simulink model "closedLoop"  (R2014b)
settings: Solver=ode45  StartTime=0.0  StopTime=inf  RelTol=1e-3
libraries: simulink x3, aerolibanimutils x1
settings Model: Creator=Owen  LastModifiedBy=Owen
settings SFSimCC: SimUserSources=TORCSLink.c
settings RTWCC: RTWUseSimCustomCode=on  CustomSource=TORCSLink.c

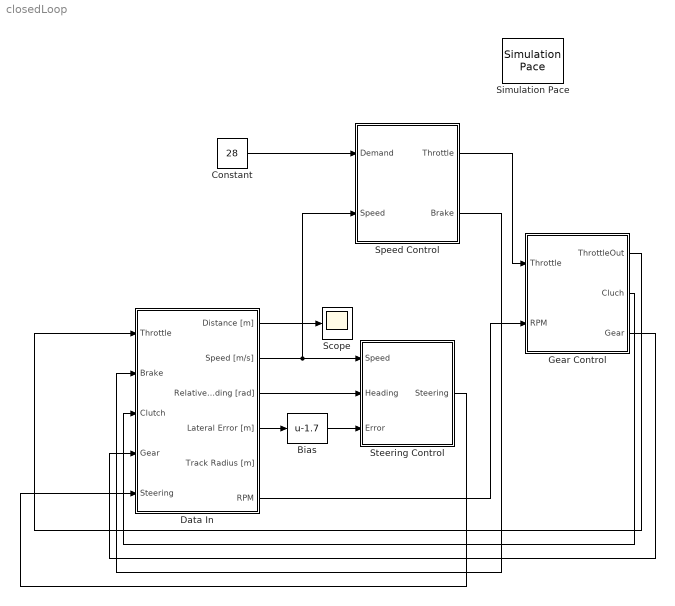
== system closedLoop ==
  Bias : Bias  Bias=-1.7
  Constant : Constant  Value=28  LockScale=on
  Data In : Subsystem
  Gear Control : Subsystem
  Scope : Scope
      settings: YMin=20250  YMax=20500  SaveName=ScopeData3
  Simulation Pace : aerolibanimutils/Simulation Pace  SimulationPace=1  SleepMode=MATLAB Thread  OutputPaceError=off  SampleTime=1/100
      settings: AttributesFormatString=%<SimulationPace> sec/sec
  Speed Control : Subsystem
  Steering Control : Subsystem
  wires:
  Data In/2(Speed [m/s]) -> Speed Control/2(Speed), Steering Control/1(Speed)
  Data In/3(Relative Heading [rad]) -> Steering Control/2(Heading)
  Data In/4(Lateral Error [m]) -> Bias/1
  Constant/1 -> Speed Control/1(Demand)
  Speed Control/1(Throttle) -> Gear Control/1(Throttle)
  Speed Control/2(Brake) -> Data In/2(Brake)
  Steering Control/1(Steering) -> Data In/5(Steering)
  Gear Control/1(ThrottleOut) -> Data In/1(Throttle)
  Gear Control/2(Cluch) -> Data In/3(Clutch)
  Gear Control/3(Gear) -> Data In/4(Gear)
  Data In/6(RPM) -> Gear Control/2(RPM)
  Bias/1 -> Steering Control/3(Error)
  Data In/1(Distance [m]) -> Scope/1

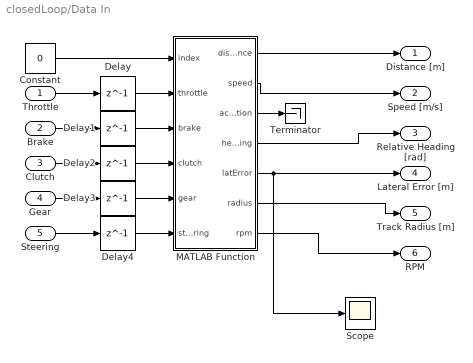
== system closedLoop/Data In ==
  Throttle : Inport
  Brake : Inport  Port=2
  Clutch : Inport  Port=3
  Gear : Inport  Port=4
  Steering : Inport  Port=5
  Constant : Constant  Value=0
  Delay{,1..4} (5 alike) : Delay  DelayLength=1  InitialCondition=0
  MATLAB Function : MATLAB Function  TreatAsAtomicUnit=on
  Scope : Scope
      settings: YMin=0.5  YMax=3  SaveName=ScopeData4
  Terminator : Terminator
  Distance [m] : Outport
  Speed [m/s] : Outport  Port=2
  Relative Heading [rad] : Outport  Port=3
  Lateral Error [m] : Outport  Port=4
  Track Radius [m] : Outport  Port=5
  RPM : Outport  Port=6
  wires:
  MATLAB Function/4(heading) -> Relative Heading [rad]/1
  MATLAB Function/2(speed) -> Speed [m/s]/1
  MATLAB Function/5(latError) -> Scope/1, Lateral Error [m]/1
  MATLAB Function/6(radius) -> Track Radius [m]/1
  MATLAB Function/1(distance) -> Distance [m]/1
  MATLAB Function/3(acceleration) -> Terminator/1
  MATLAB Function/7(rpm) -> RPM/1
  Constant/1 -> MATLAB Function/1(index)
  Brake/1 -> Delay1/1
  Clutch/1 -> Delay2/1
  Gear/1 -> Delay3/1
  Steering/1 -> Delay4/1
  Delay/1 -> MATLAB Function/2(throttle)
  Delay1/1 -> MATLAB Function/3(brake)
  Delay2/1 -> MATLAB Function/4(clutch)
  Delay3/1 -> MATLAB Function/5(gear)
  Delay4/1 -> MATLAB Function/6(steering)
  Throttle/1 -> Delay/1

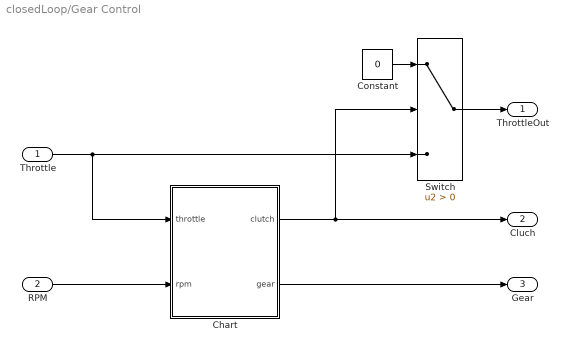
== system closedLoop/Gear Control ==
  Throttle : Inport
  RPM : Inport  Port=2
  Chart : Stateflow chart  TreatAsAtomicUnit=on
  Constant : Constant  Value=0  OutDataTypeStr=single
  Switch : Switch  Criteria=u2 > Threshold
  ThrottleOut : Outport
  Cluch : Outport  Port=2
  Gear : Outport  Port=3
  wires:
  Chart/1(clutch) -> Switch/2, Cluch/1
  Chart/2(gear) -> Gear/1
  Switch/1 -> ThrottleOut/1
  Constant/1 -> Switch/1
  RPM/1 -> Chart/2(rpm)
  Throttle/1 -> Chart/1(throttle), Switch/3

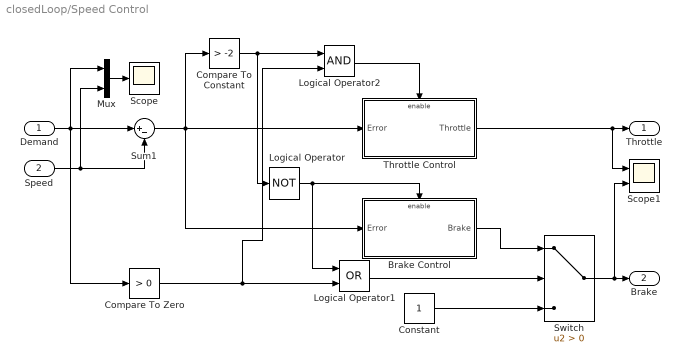
== system closedLoop/Speed Control ==
  Demand : Inport
  Speed : Inport  Port=2
  Brake Control : Subsystem
  Compare To Constant : simulink/Logic and Bit Operations/Compare To Constant  relop=>  const=-2  OutDataTypeStr=boolean
  Compare To Zero : simulink/Logic and Bit Operations/Compare To Zero  relop=>  OutDataTypeStr=boolean
  Constant : Constant  OutDataTypeStr=single
  Logical Operator : Logic  Operator=NOT  AllPortsSameDT=off  OutDataTypeStr=boolean
  Logical Operator1 : Logic  Operator=OR  AllPortsSameDT=off  OutDataTypeStr=boolean
  Logical Operator2 : Logic  AllPortsSameDT=off  OutDataTypeStr=boolean
  Mux : Mux  Inputs=2
  Scope : Scope
      settings: YMin=27.8  YMax=28.2
  Scope1 : Scope  NumInputPorts=2
      settings: YMin=-0~-0  YMax=2~2  SaveName=ScopeData2
  Sum1 : Sum  Inputs=|+-
  Switch : Switch  Criteria=u2 > Threshold
  Throttle Control : Subsystem
  Throttle : Outport
  Brake : Outport  Port=2
  wires:
  Speed/1 -> Sum1/2, Mux/2
  Mux/1 -> Scope/1
  Demand/1 -> Compare To Zero/1, Sum1/1, Mux/1
  Sum1/1 -> Brake Control/1(Error), Compare To Constant/1, Throttle Control/1(Error)
  Throttle Control/1(Throttle) -> Scope1/1, Throttle/1
  Compare To Constant/1 -> Logical Operator2/1, Logical Operator/1
  Logical Operator/1 -> Logical Operator1/1, Brake Control/Enable
  Switch/1 -> Scope1/2, Brake/1
  Brake Control/1(Brake) -> Switch/1
  Constant/1 -> Switch/3
  Compare To Zero/1 -> Logical Operator2/2, Logical Operator1/2
  Logical Operator1/1 -> Switch/2
  Logical Operator2/1 -> Throttle Control/Enable

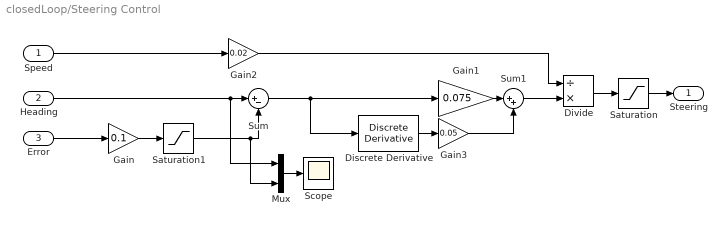
== system closedLoop/Steering Control ==
  Speed : Inport
  Heading : Inport  Port=2
  Error : Inport  Port=3
  Discrete Derivative : simulink/Discrete/Discrete Derivative  gainval=1.0  ICPrevScaledInput=0.0  InputProcessing=Inherited  OutMin=[]  OutMax=[]  OutDataType=fixdt(1, 16)  OutScaling=2^-10  DoSatur=off
  Divide : Product  Inputs=/*
  Gain : Gain  Gain=0.1
  Gain1 : Gain  Gain=0.075
  Gain2 : Gain  Gain=0.02
  Gain3 : Gain  Gain=0.05
  Mux : Mux  Inputs=2
  Saturation : Saturate
  Saturation1 : Saturate  UpperLimit=0.2  LowerLimit=-0.2
  Scope : Scope
      settings: YMin=-0.3  YMax=0.2
  Sum : Sum  Inputs=|+-
  Sum1 : Sum  Inputs=|++
  Steering : Outport
  wires:
  Heading/1 -> Mux/1, Sum/1
  Error/1 -> Gain/1
  Speed/1 -> Gain2/1
  Gain2/1 -> Divide/1
  Sum/1 -> Discrete Derivative/1, Gain1/1
  Gain/1 -> Saturation1/1
  Divide/1 -> Saturation/1
  Gain1/1 -> Sum1/1
  Saturation/1 -> Steering/1
  Mux/1 -> Scope/1
  Discrete Derivative/1 -> Gain3/1
  Sum1/1 -> Divide/2
  Gain3/1 -> Sum1/2
  Saturation1/1 -> Mux/2, Sum/2

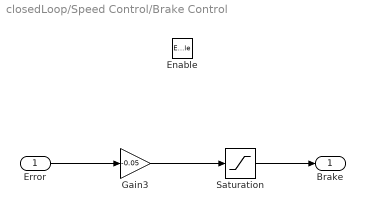
== system closedLoop/Speed Control/Brake Control ==
  Error : Inport
  Enable : EnablePort
  Gain3 : Gain  Gain=-0.05
  Saturation : Saturate  LowerLimit=0
  Brake : Outport  OutputWhenDisabled=reset  InitialOutput=0
  wires:
  Gain3/1 -> Saturation/1
  Saturation/1 -> Brake/1
  Error/1 -> Gain3/1

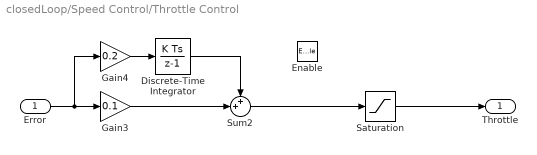
== system closedLoop/Speed Control/Throttle Control ==
  Error : Inport
  Enable : EnablePort
  Discrete-Time Integrator : DiscreteIntegrator  InitialConditionSetting=State (most efficient)  SampleTime=-1  LimitOutput=on  UpperSaturationLimit=0.5  LowerSaturationLimit=-0.5
  Gain3 : Gain  Gain=0.1
  Gain4 : Gain  Gain=0.2
  Saturation : Saturate  UpperLimit=1  LowerLimit=0
  Sum2 : Sum  Inputs=++|
  Throttle : Outport  OutputWhenDisabled=reset  InitialOutput=0
  wires:
  Discrete-Time Integrator/1 -> Sum2/1
  Error/1 -> Gain4/1, Gain3/1
  Saturation/1 -> Throttle/1
  Gain4/1 -> Discrete-Time Integrator/1
  Sum2/1 -> Saturation/1
  Gain3/1 -> Sum2/2

== stateflow chart closedLoop/Gear Control/Chart ==
  state ShiftLogic [parallel]
    en: gear = int32(1); minRPM = 2000; maxRPM = 6000;
    settings: executionOrder=1
    state Downshift
      en:clutch = single(1);
      ex: gear = gear - int32(1);
    state SteadyState
      en: clutch =single(0);
    state Upshift
      en: clutch = single(1);
      ex: gear = gear + int32(1);
    (default) -> SteadyState
    SteadyState -> Upshift [order 1] : after(100,msec)[gear < 5 && (rpm > maxRPM || (throttle < 0.25 && rpm > minRPM))]
    SteadyState -> Downshift [order 2] : after(100,msec)[throttle > 0.25 && (gear > 1 && rpm < minRPM)]
    Upshift -> SteadyState : after(100,msec)
    Downshift -> SteadyState : after(100,msec)
  data: throttle input; rpm input; clutch output single; minRPM local; maxRPM local; gear output int32

== matlab function closedLoop/Data In/MATLAB Function ==
  data: distance output; index input; throttle input; brake input; clutch input; gear input; steering input; speed output; acceleration output; heading output; latError output; radius output; rpm output
function ...
    [distance, speed, acceleration, heading, latError, radius, rpm] = ...
    UpdateVehicle(index, throttle,brake,clutch,gear,steering)
%#codegen

veh = struct( ...
    'throttle', single(0),...
    'brake', single(0),...
    'clutch', single(0),...
    'steering', single(0),...
    'gear', int32(0),...
    'dist', single(0),...
    'speed', single(0),...
    'accel', single(0),...
    'angle', single(0),...
    'latErr', single(0),...
    'radius', single(0),...
    'rpm', single(0));

% Assign our outputs
veh.throttle = single(throttle);
veh.brake = single(brake);
veh.clutch = single(clutch);
veh.steering = single(steering);
veh.gear = int32(gear);


% Synchronise with TORCS
coder.ceval('updateVehicle', int32(index), coder.ref(veh));

% Update outputs
distance = double(veh.dist);
speed = double(veh.speed);
acceleration = double(veh.accel);
heading = double(veh.angle);
latError = double(veh.latErr);
radius = double(veh.radius);
rpm = double(veh.rpm);
